simulink model "APP_Coherency"  (R2022b)
settings: Solver=VariableStepAuto  StartTime=0.0  StopTime=10.0  RelTol=1e-3
settings Model: Creator=ahmed  LastModifiedBy=ahmed

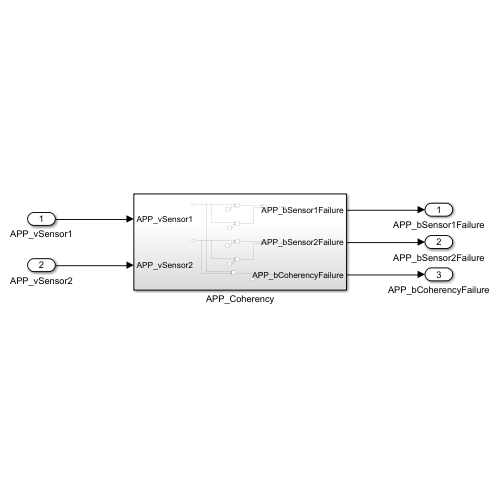
[thumbnail: Simulink's stored preview of the top-level diagram]
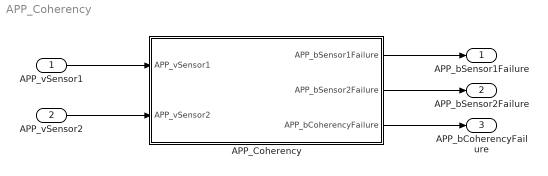
== system APP_Coherency ==
  APP_vSensor1 : Inport
  APP_vSensor2 : Inport  Port=2
  APP_Coherency : Subsystem
  APP_bSensor1Failure : Outport
  APP_bSensor2Failure : Outport  Port=2
  APP_bCoherencyFailure : Outport  Port=3
  wires:
  APP_Coherency/1(APP_bSensor1Failure) -> APP_bSensor1Failure/1
  APP_Coherency/2(APP_bSensor2Failure) -> APP_bSensor2Failure/1
  APP_Coherency/3(APP_bCoherencyFailure) -> APP_bCoherencyFailure/1
  APP_vSensor1/1 -> APP_Coherency/1(APP_vSensor1)
  APP_vSensor2/1 -> APP_Coherency/2(APP_vSensor2)

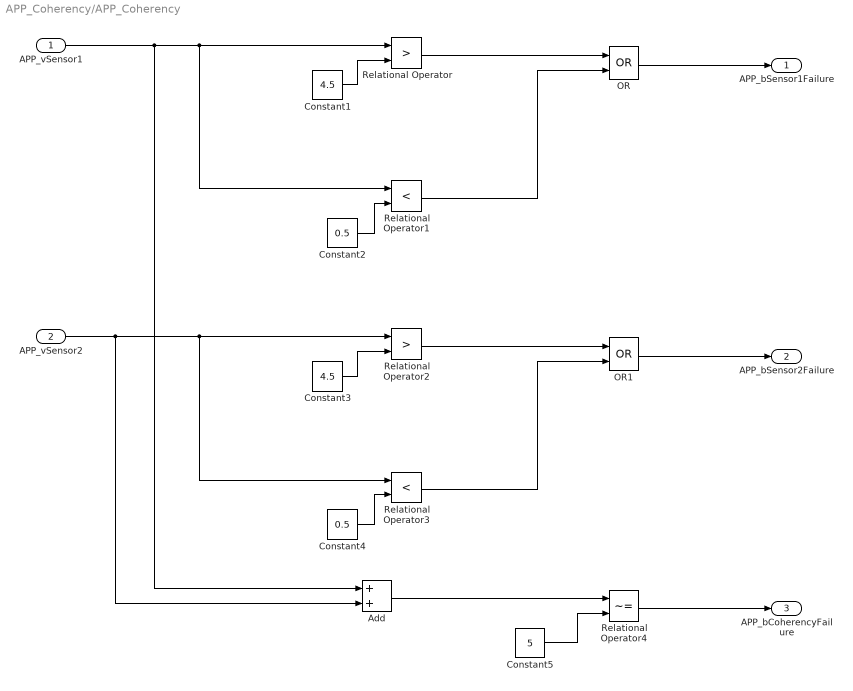
== system APP_Coherency/APP_Coherency ==
  APP_vSensor1 : Inport
  APP_vSensor2 : Inport  Port=2
  Add : Sum
  Constant1 : Constant  Value=4.5
  Constant2 : Constant  Value=0.5
  Constant3 : Constant  Value=4.5
  Constant4 : Constant  Value=0.5
  Constant5 : Constant  Value=5
  OR : Logic  Operator=OR  AllPortsSameDT=off  OutDataTypeStr=boolean
  OR1 : Logic  Operator=OR  AllPortsSameDT=off  OutDataTypeStr=boolean
  Relational Operator : RelationalOperator  Operator=>  OutDataTypeStr=boolean  RndMeth=Simplest  InputSameDT=off
  Relational Operator1 : RelationalOperator  Operator=<  OutDataTypeStr=boolean  RndMeth=Simplest  InputSameDT=off
  Relational Operator2 : RelationalOperator  Operator=>  OutDataTypeStr=boolean  RndMeth=Simplest  InputSameDT=off
  Relational Operator3 : RelationalOperator  Operator=<  OutDataTypeStr=boolean  RndMeth=Simplest  InputSameDT=off
  Relational Operator4 : RelationalOperator  Operator=~=  OutDataTypeStr=boolean  RndMeth=Simplest  InputSameDT=off
  APP_bSensor1Failure : Outport
  APP_bSensor2Failure : Outport  Port=2
  APP_bCoherencyFailure : Outport  Port=3
  wires:
  Relational Operator4/1 -> APP_bCoherencyFailure/1
  APP_vSensor1/1 -> Relational Operator1/1, Relational Operator/1, Add/1
  Constant5/1 -> Relational Operator4/2
  OR/1 -> APP_bSensor1Failure/1
  Relational Operator1/1 -> OR/2
  Constant4/1 -> Relational Operator3/2
  Constant1/1 -> Relational Operator/2
  OR1/1 -> APP_bSensor2Failure/1
  Constant2/1 -> Relational Operator1/2
  Add/1 -> Relational Operator4/1
  Relational Operator2/1 -> OR1/1
  Relational Operator/1 -> OR/1
  APP_vSensor2/1 -> Relational Operator3/1, Relational Operator2/1, Add/2
  Constant3/1 -> Relational Operator2/2
  Relational Operator3/1 -> OR1/2
